simulink model "Outputs"  (R2018b)
settings: configuration reference "FixedStepConfiguration" (kept outside this file)
libraries: arduinolib x2
settings Model: DataDictionary=DataDictionary.sldd  Creator=chris  LastModifiedBy=chris

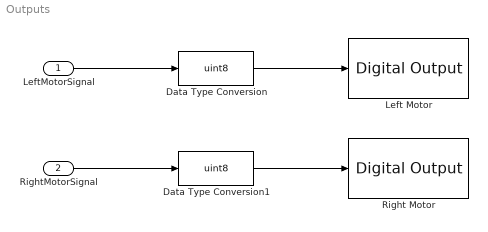
== system Outputs ==
  LeftMotorSignal : Inport  OutDataTypeStr=double
  RightMotorSignal : Inport  Port=2  OutDataTypeStr=double
  Data Type Conversion : DataTypeConversion  OutDataTypeStr=uint8
  Data Type Conversion1 : DataTypeConversion  OutDataTypeStr=uint8
  Left Motor : arduinolib/Digital Output  pinNumber=4  blockPlatform=arduino
  Right Motor : arduinolib/Digital Output  pinNumber=4  blockPlatform=arduino
  wires:
  LeftMotorSignal/1 -> Data Type Conversion/1
  RightMotorSignal/1 -> Data Type Conversion1/1
  Data Type Conversion/1 -> Left Motor/1
  Data Type Conversion1/1 -> Right Motor/1
